simulink model "I4_11_3_kinect_Simulink"  (R2014a)
settings: Solver=FixedStepDiscrete  SolverMode=SingleTasking  StartTime=0.0  StopTime=Inf  RelTol=1e-3
values from neighbouring files (symbols this model uses):
  C = imread('cameraman.tif')    [I2_01_2_display_investigation.m]    (also in I2_01_4_graphics.m = convexHull(DT))
undefined symbols (not defined in the file or in its folder): IsPositionTracked, IsSkeletonTracked, JointDepthIndices, JointImageIndices, JointTrackingState, JointWorldCoordinates, none, PositionDepthIndices, PositionImageIndices, PositionWorldCoordinates, SegmentationData, SkeletonTrackingID, videoinput
libraries: visiontextngfix x4, visionsinks x3, imaqlib x2
settings Model: Creator=motobe  LastModifiedBy=motobe
settings DataIOCC: SignalLogging=off
settings OptimizationCC: BlockReduction=off  ConditionallyExecuteInputs=off  InlineParams=on  OptimizeModelRefInitCode=on  LifeSpan=Inf
settings DebuggingCC: AlgebraicLoopMsg=error  UnderspecifiedInitializationDetection=Classic  SingleTaskRateTransMsg=error
settings HardwareCC: ProdBitPerInt=16  ProdBitPerPointer=16  ProdWordSize=16  ProdHWDeviceType=Generic->16-bit Embedded Processor  TargetLongLongMode=on  TargetIntDivRoundTo=Zero  TargetEndianess=LittleEndian  TargetHWDeviceType=MATLAB Host  ProdEqTarget=off
settings RTWCC: SystemTargetFile=ert.tlc  TemplateMakefile=ert_default_tmf  Description=Embedded Coder  GenerateReport=on  ProcessScript=ert_make_rtw_hook  IncludeHyperlinkInReport=on  LaunchReport=on
settings CodeAppCC: IgnoreCustomStorageClasses=off
settings ERTTargetCC: ParMdlRefBuildCompliant=on  CompOptLevelCompliant=on  ConcurrentExecutionCompliant=on  ERTFirstTimeCompliant=on  ModelStepFunctionPrototypeControlCompliant=on  CPPClassGenCompliant=on  ERTCustomFileTemplate=example_file_process.tlc

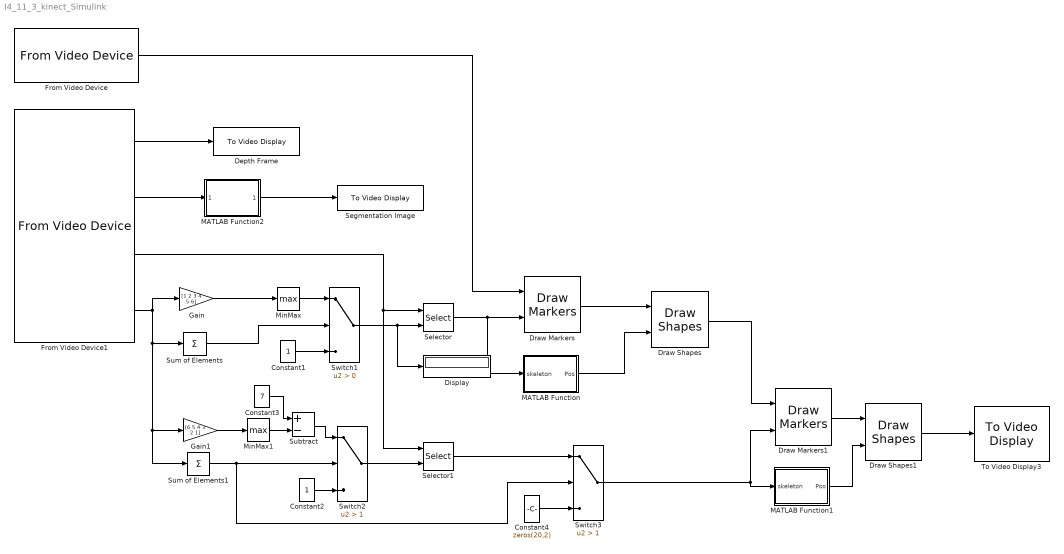
== system I4_11_3_kinect_Simulink ==
  Constant1 : Constant  OutDataTypeStr=uint8  SampleTime=Inf
  Constant2 : Constant  OutDataTypeStr=uint8  SampleTime=Inf
  Constant3 : Constant  Value=7  OutDataTypeStr=uint8  SampleTime=Inf
  Constant4 : Constant  Value=zeros(20,2)  OutDataTypeStr=uint8  SampleTime=Inf
  Depth Frame : visionsinks/To Video Display  inputType=Obsolete  imagePorts=One multidimensional signal  OutputDevice=On-screen video monitor  fullScreen=off  videoWindowX=1314  videoWindowY=206  saveWindowSize=off  videoWindowWidth=373  videoWindowHeight=296  dataOrg=Column-major  openAtMdlStart=on  isWindowOpen=on  inputColorFormat=RGB
  Display : Display
  Draw Markers : visiontextngfix/Draw Markers  shape=Circle  size=5  fill=on  fillClrSource=Specify via dialog  display=User-specified value  intensity=200  color=[255 255 0]  opacity=0.6  viewport=Entire image  antialiasing=off  inType=Obsolete  imagePorts=One multidimensional signal  prodOutputMode=Binary point scaling  prodOutputWordLength=32  prodOutputFracLength=14  memoryMode=Specify word length  memoryWordLength=16  memoryFracLength=14  roundingMode=Floor  overflowMode=off
  Draw Markers1 : visiontextngfix/Draw Markers  shape=Circle  size=5  fill=on  fillClrSource=Specify via dialog  display=User-specified value  intensity=200  color=[255 0 0]  opacity=0.6  viewport=Entire image  antialiasing=off  inType=Obsolete  imagePorts=One multidimensional signal  prodOutputMode=Binary point scaling  prodOutputWordLength=32  prodOutputFracLength=14  memoryMode=Specify word length  memoryWordLength=16  memoryFracLength=14  roundingMode=Floor  overflowMode=off
  Draw Shapes : visiontextngfix/Draw Shapes  shape=Lines  fill=off  lineWidth=3  fillClrSource=Specify via dialog  display=User-specified value  intensity=200  color=[255 255 0]  opacity=0.6  viewport=Entire image  antialiasing=off  inType=Obsolete  imagePorts=One multidimensional signal  prodOutputMode=Binary point scaling  prodOutputWordLength=32  prodOutputFracLength=14  memoryMode=Specify word length  memoryWordLength=16  memoryFracLength=14  roundingMode=Floor  overflowMode=off
  Draw Shapes1 : visiontextngfix/Draw Shapes  shape=Lines  fill=off  lineWidth=3  fillClrSource=Specify via dialog  display=User-specified value  intensity=200  color=[255 0 0]  opacity=0.6  viewport=Entire image  antialiasing=off  inType=Obsolete  imagePorts=One multidimensional signal  prodOutputMode=Binary point scaling  prodOutputWordLength=32  prodOutputFracLength=14  memoryMode=Specify word length  memoryWordLength=16  memoryFracLength=14  roundingMode=Floor  overflowMode=off
  From Video Device : imaqlib/From Video Device  DeviceMenu=kinect 1 (Kinect Color Sensor)  Device=kinect 1 (Kinect Color Sensor)  ObjConstructor=videoinput('kinect', 1)  VideoFormatMenu=RGB_640x480  VideoFormat=RGB_640x480  VideoSource=Color Source  ROIPosition=[0 0 480 640]  EnableHWTrigger=off  TriggerConfiguration=none/none  SampleTime=1/30  OutputPortsMode=One multidimensional signal  DataType=single  CanDoHWTrigger=no  ReturnedColorSpace=rgb  BlockHandle=1914.0001  ROIWidth=640  ROIHeight=480  ROIColumn=0  ROIRow=0  EngXMLPath=C:\MATLAB\R2014a\toolbox\imaq\imaq\private  DevXMLPath=C:\MATLAB\SupportPackages\R2014a\kinectruntime\adaptor\win64  EngLibPath=C:\MATLAB\R2014a\toolbox\imaq\imaqblks\imaqmex\win64  ColorSpace=rgb  BayerSensorAlignment=grbg  AllMetadata=IsPositionTracked;IsSkeletonTracked;JointDepthIndices;JointImageIndices;JointTrackingState;JointWorldCoordinates;PositionDepthIndices;PositionImageIndices;PositionWorldCoordinates;SegmentationData;SkeletonTrackingID
  From Video Device1 : imaqlib/From Video Device  DeviceMenu=kinect 2 (Kinect Depth Sensor)  Device=kinect 2 (Kinect Depth Sensor)  ObjConstructor=videoinput('kinect', 2)  VideoFormatMenu=Depth_640x480  VideoFormat=Depth_640x480  VideoSource=Depth Source  ROIPosition=[0 0 480 640]  EnableHWTrigger=off  TriggerConfiguration=none/none  SampleTime=1/30  OutputPortsMode=One multidimensional signal  DataType=single  CanDoHWTrigger=no  ReturnedColorSpace=grayscale  BlockHandle=1914.0001  ROIWidth=640  ROIHeight=480  ROIColumn=0  ROIRow=0  EngXMLPath=C:\MATLAB\R2014a\toolbox\imaq\imaq\private  DevXMLPath=C:\MATLAB\SupportPackages\R2014a\kinectruntime\adaptor\win64  EngLibPath=C:\MATLAB\R2014a\toolbox\imaq\imaqblks\imaqmex\win64  ColorSpace=grayscale  BayerSensorAlignment=grbg  AllMetadata=IsPositionTracked;IsSkeletonTracked;JointDepthIndices;JointImageIndices;JointTrackingState;JointWorldCoordinates;PositionDepthIndices;PositionImageIndices;PositionWorldCoordinates;SegmentationData;SkeletonTrackingID  SelectedMetadata=SegmentationData;JointImageIndices;IsSkeletonTracked
  Gain : Gain  Gain=[1 2 3 4 5 6]  OutDataTypeStr=uint8
  Gain1 : Gain  Gain=[6 5 4 3 2 1]  OutDataTypeStr=uint8
  MATLAB Function : MATLAB Function  TreatAsAtomicUnit=on
  MATLAB Function1 : MATLAB Function  TreatAsAtomicUnit=on
  MATLAB Function2 : MATLAB Function  TreatAsAtomicUnit=on
  MinMax : MinMax  Function=max
  MinMax1 : MinMax  Function=max
  Segmentation Image : visionsinks/To Video Display  inputType=Obsolete  imagePorts=One multidimensional signal  OutputDevice=On-screen video monitor  fullScreen=off  videoWindowX=1315  videoWindowY=595  saveWindowSize=off  videoWindowWidth=375  videoWindowHeight=290  dataOrg=Column-major  openAtMdlStart=on  isWindowOpen=on  inputColorFormat=RGB
  Selector : Selector  NumberOfDimensions=3  InputPortWidth=3  IndexOptions=Select all,Select all,Index vector (port)  Indices=[1 3],1,1  OutputSizes=1,1,1
  Selector1 : Selector  NumberOfDimensions=3  InputPortWidth=3  IndexOptions=Select all,Select all,Index vector (port)  Indices=[1 3],1,1  OutputSizes=1,1,1
  Subtract : Sum  Inputs=+-
  Sum of Elements : Sum  Inputs=+  AccumDataTypeStr=uint8
  Sum of Elements1 : Sum  Inputs=+  AccumDataTypeStr=uint8
  Switch1 : Switch  Criteria=u2 > Threshold
  Switch2 : Switch  Criteria=u2 > Threshold  Threshold=1
  Switch3 : Switch  Criteria=u2 > Threshold  Threshold=1
  To Video Display3 : visionsinks/To Video Display  inputType=Obsolete  imagePorts=One multidimensional signal  OutputDevice=On-screen video monitor  fullScreen=off  videoWindowX=684  videoWindowY=210  saveWindowSize=off  videoWindowWidth=441  videoWindowHeight=300  dataOrg=Column-major  openAtMdlStart=on  isWindowOpen=on  inputColorFormat=RGB
  wires:
  From Video Device/1 -> Draw Markers/1
  From Video Device1/1 -> Depth Frame/1
  From Video Device1/2 -> MATLAB Function2/1(SegmentationData)
  From Video Device1/3 -> Selector1/1, Selector/1
  Switch1/1 -> Display/1, Selector/2
  Selector/1 -> MATLAB Function/1(skeleton), Draw Markers/2
  Draw Shapes/1 -> Draw Markers1/1
  Gain/1 -> MinMax/1
  Draw Markers/1 -> Draw Shapes/1
  MATLAB Function/1(Pos) -> Draw Shapes/2
  From Video Device1/4 -> Sum of Elements1/1, Gain1/1, Sum of Elements/1, Gain/1
  Gain1/1 -> MinMax1/1
  Switch2/1 -> Selector1/2
  Switch3/1 -> Draw Markers1/2, MATLAB Function1/1(skeleton)
  Draw Markers1/1 -> Draw Shapes1/1
  MATLAB Function1/1(Pos) -> Draw Shapes1/2
  Draw Shapes1/1 -> To Video Display3/1
  MinMax/1 -> Switch1/1
  Sum of Elements/1 -> Switch1/2
  Constant1/1 -> Switch1/3
  MinMax1/1 -> Subtract/2
  Constant3/1 -> Subtract/1
  MATLAB Function2/1(SegRGB) -> Segmentation Image/1
  Subtract/1 -> Switch2/1
  Sum of Elements1/1 -> Switch2/2, Switch3/2
  Selector1/1 -> Switch3/1
  Constant2/1 -> Switch2/3
  Constant4/1 -> Switch3/3

== matlab function I4_11_3_kinect_Simulink/MATLAB Function1 ==
  data: skeleton input; Pos output
function Pos = fcn(skeleton)
%#codegen

SkeletonConnectionMap = [[1 2];
                         [2 3];
                         [3 4];
                         [3 5];
                         [5 6];
                         [6 7];
                         [7 8];
                         [3 9];
                         [9 10];
                         [10 11];
                         [11 12];
                         [1 17];
                         [17 18];
                         [18 19];
                         [19 20];
                         [1 13];
                         [13 14];
                         [14 15];
                         [15 16]];
 
Pos = zeros(19,4);

for i = 1:19
    Pos(i,:) = [skeleton(SkeletonConnectionMap(i,1),1,1) skeleton(SkeletonConnectionMap(i,1),2,1) ...
                 skeleton(SkeletonConnectionMap(i,2),1,1) skeleton(SkeletonConnectionMap(i,2),2,1)];
end

== matlab function I4_11_3_kinect_Simulink/MATLAB Function ==
  data: skeleton input; Pos output
function Pos = fcn(skeleton)
%#codegen

SkeletonConnectionMap = [[1 2];
                         [2 3];
                         [3 4];
                         [3 5];
                         [5 6];
                         [6 7];
                         [7 8];
                         [3 9];
                         [9 10];
                         [10 11];
                         [11 12];
                         [1 17];
                         [17 18];
                         [18 19];
                         [19 20];
                         [1 13];
                         [13 14];
                         [14 15];
                         [15 16]];
 
Pos = zeros(19,4);

for i = 1:19
    Pos(i,:) = [skeleton(SkeletonConnectionMap(i,1),1,1) skeleton(SkeletonConnectionMap(i,1),2,1) ...
                 skeleton(SkeletonConnectionMap(i,2),1,1) skeleton(SkeletonConnectionMap(i,2),2,1)];
end

== matlab function I4_11_3_kinect_Simulink/MATLAB Function2 ==
  data: SegmentationData input; SegRGB output size=[480 640 3]
function SegRGB = fcn(SegmentationData)
%#codegen
cmap = [ ...
         0         0    0.7500; ...
         0         0    1.0000; ...
         0    0.2500    1.0000; ...
         0    0.5000    1.0000; ...
         0    0.7500    1.0000; ...
         0    1.0000    1.0000; ...
    0.2500    1.0000    0.7500; ...
    0.5000    1.0000    0.5000; ...
    0.7500    1.0000    0.2500; ...
    1.0000    1.0000         0; ...
    1.0000    0.7500         0; ...
    1.0000    0.5000         0; ...
    1.0000    0.2500         0; ...
    1.0000         0         0; ...
    0.7500         0         0; ...
    0.5000         0         0];


SegRGB = label2rgb(SegmentationData, cmap,'k');
